simulink model "untitled"  (R2019b)
settings: Solver=VariableStepAuto  StartTime=0.0  StopTime=10.0  RelTol=1e-3
undefined symbols (not defined in the file): m, n
settings Model: Creator=Εμμανουήλ  LastModifiedBy=Εμμανουήλ

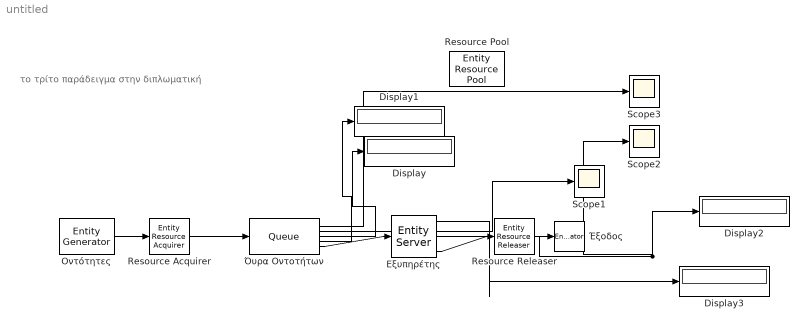
== system untitled ==
  note: το τρίτο παράδειγμα στην διπλωματική
  Display{,1..3} (4 alike) : Display
  Resource Acquirer : EntityResourceAcquirer  InputPortMessageModes=m  OutputPortMessageModes=m
      settings: OutputPortMap=o3
  Resource Releaser : EntityResourceReleaser  InputPortMessageModes=m  OutputPortMessageModes=m
  Resource Pool : EntityResourcePool
  Scope1 : Scope
  Scope2 : Scope
  Scope3 : Scope
  Έξοδος : EntityTerminator  InputPortMessageModes=m
  Όυρα Οντοτήτων : Queue  InputPortMessageModes=m  OutputPortMessageModes=n,n,n,n,m  NumberEntitiesDeparted=on  NumberEntitiesInBlock=on  AverageWait=on  AverageQueueLength=on
      settings: OutputPortMap=o0,o1,o2,o3,o5
  Εξυπηρέτης : EntityServer  InputPortMessageModes=m  OutputPortMessageModes=n,n,m  Capacity=1  ServiceTimeSource=MATLAB action  ServiceTimeAction=|  AverageWait=on  Utilization=on
      | persistent rngInit;
      | if isempty(rngInit)
      |     seed = 12345;
      |     rng(seed);
      |     rngInit = true;
      | end
      | 
      | % Pattern: Poisson distribution
      | % m: Mean
      | m = 5;
      | dt = poissrnd(m);
      settings: OutputPortMap=o4,o5,o9
  Οντότητες : EntityGenerator  OutputPortMessageModes=m  TimeSource=MATLAB action  IntergenerationTimeAction=|  EntityType=Structured  EntityTypeName=Entity
      | % Pattern: Repeating Sequence
      | persistent SEQ;
      | persistent idx;
      | if isempty(SEQ)
      |     SEQ = [zeros(1,10) 1000];
      |     idx = 1;
      | end
      | dt = idx;
      | dt = SEQ(idx);
      | idx = idx + 1;
  wires:
  Όυρα Οντοτήτων/4 -> Display1/1
  Όυρα Οντοτήτων/1 -> Scope3/1
  Οντότητες/1 -> Resource Acquirer/1
  Εξυπηρέτης/3 -> Resource Releaser/1
  Resource Acquirer/1 -> Όυρα Οντοτήτων/1
  Εξυπηρέτης/1 -> Display3/1
  Εξυπηρέτης/2 -> Scope2/1, Display2/1
  Όυρα Οντοτήτων/3 -> Display/1
  Όυρα Οντοτήτων/2 -> Scope1/1
  Resource Releaser/1 -> Έξοδος/1
  Όυρα Οντοτήτων/5 -> Εξυπηρέτης/1
